simulink model "simulacija"  (R2015a)
settings: Solver=ode45  StartTime=0.0  StopTime=500  RelTol=1e-3
values from neighbouring files (symbols this model uses):
  C = C_r/m    (= 5.618808)    [parametri.m]
  K = 2*n*R_t/R    [parametri.m]
  R = R_r/m    [parametri.m]
  R_s1 = 1/(alfa_vaz*2*(a+b)*L/m)    (= 89.1265597148)    [parametri.m]
  R_s2 = 1/(alfa_vaz*a*b)    (= 1014.19878296)    [parametri.m]
  teta_k = 70    [parametri.m]
  teta_vaz = 30    [parametri.m]
settings Model: Creator=zracenje  LastModifiedBy=Danijel
settings DebuggingCC: UnderspecifiedInitializationDetection=Classic  MergeDetectMultiDrivingBlocksExec=none  SolverPrmCheckMsg=warning

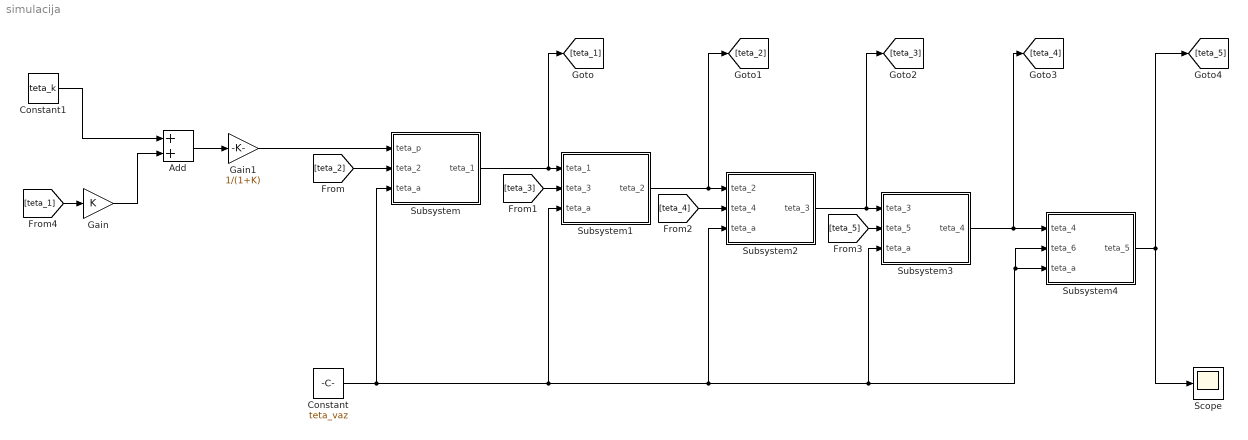
== system simulacija ==
  Add : Sum
  Constant : Constant  Value=teta_vaz
  Constant1 : Constant  Value=teta_k
  Gain : Gain  Gain=K
  Gain1 : Gain  Gain=1/(1+K)
  Scope : Scope
      settings: TimeRange=500  YMin=30  YMax=65
  Subsystem : Subsystem
  Subsystem1 : Subsystem
  Subsystem2 : Subsystem
  Subsystem3 : Subsystem
  Subsystem4 : Subsystem
  wires:
  Subsystem/1(teta_1) -> [teta_1], Subsystem1/1(teta_1)
  Subsystem1/1(teta_2) -> [teta_2], Subsystem2/1(teta_2)
  Subsystem2/1(teta_3) -> [teta_3], Subsystem3/1(teta_3)
  Subsystem3/1(teta_4) -> [teta_4], Subsystem4/1(teta_4)
  Constant/1 -> Subsystem1/3("teta_a "), Subsystem2/3("teta_a "), Subsystem3/3("teta_a "), Subsystem4/2(teta_6), Subsystem4/3("teta_a "), Subsystem/3("teta_a ")
  Subsystem4/1(teta_5) -> [teta_5], Scope/1
  [teta_2] -> Subsystem/2(teta_2)
  [teta_3] -> Subsystem1/2(teta_3)
  [teta_4] -> Subsystem2/2(teta_4)
  [teta_5] -> Subsystem3/2(teta_5)
  Constant1/1 -> Add/1
  Gain/1 -> Add/2
  [teta_1] -> Gain/1
  Add/1 -> Gain1/1
  Gain1/1 -> Subsystem/1(teta_p)

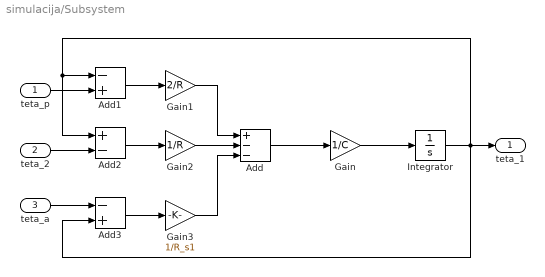
== system simulacija/Subsystem ==
  teta_p : Inport
  teta_2 : Inport  Port=2
  "teta_a " : Inport  Port=3
  Add : Sum  Inputs=+--
  Add1 : Sum  Inputs=-+
  Add2 : Sum  Inputs=+-
  Add3 : Sum  Inputs=-+
  Gain : Gain  Gain=1/C
  Gain1 : Gain  Gain=2/R
  Gain2 : Gain  Gain=1/R
  Gain3 : Gain  Gain=1/R_s1
  Integrator : Integrator  InitialCondition=teta_vaz
  teta_1 : Outport
  wires:
  Add/1 -> Gain/1
  Gain/1 -> Integrator/1
  Integrator/1 -> Add3/2, Add1/1, Add2/1, teta_1/1
  Add1/1 -> Gain1/1
  Gain1/1 -> Add/1
  Gain2/1 -> Add/2
  Add2/1 -> Gain2/1
  Gain3/1 -> Add/3
  Add3/1 -> Gain3/1
  "teta_a "/1 -> Add3/1
  teta_2/1 -> Add2/2
  teta_p/1 -> Add1/2

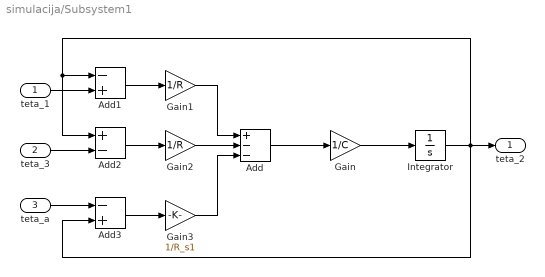
== system simulacija/Subsystem1 ==
  teta_1 : Inport
  teta_3 : Inport  Port=2
  "teta_a " : Inport  Port=3
  Add : Sum  Inputs=+--
  Add1 : Sum  Inputs=-+
  Add2 : Sum  Inputs=+-
  Add3 : Sum  Inputs=-+
  Gain : Gain  Gain=1/C
  Gain1 : Gain  Gain=1/R
  Gain2 : Gain  Gain=1/R
  Gain3 : Gain  Gain=1/R_s1
  Integrator : Integrator  InitialCondition=teta_vaz
  teta_2 : Outport
  wires:
  Add/1 -> Gain/1
  Gain/1 -> Integrator/1
  Integrator/1 -> Add3/2, Add1/1, Add2/1, teta_2/1
  Add1/1 -> Gain1/1
  Gain1/1 -> Add/1
  Gain2/1 -> Add/2
  Add2/1 -> Gain2/1
  Gain3/1 -> Add/3
  Add3/1 -> Gain3/1
  "teta_a "/1 -> Add3/1
  teta_3/1 -> Add2/2
  teta_1/1 -> Add1/2

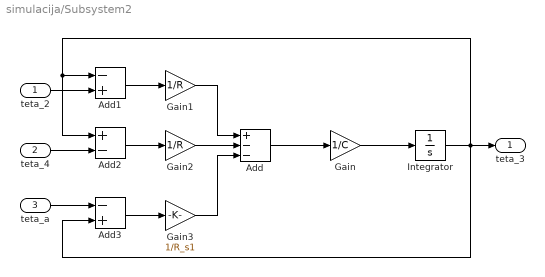
== system simulacija/Subsystem2 ==
  teta_2 : Inport
  teta_4 : Inport  Port=2
  "teta_a " : Inport  Port=3
  Add : Sum  Inputs=+--
  Add1 : Sum  Inputs=-+
  Add2 : Sum  Inputs=+-
  Add3 : Sum  Inputs=-+
  Gain : Gain  Gain=1/C
  Gain1 : Gain  Gain=1/R
  Gain2 : Gain  Gain=1/R
  Gain3 : Gain  Gain=1/R_s1
  Integrator : Integrator  InitialCondition=teta_vaz
  teta_3 : Outport
  wires:
  Add/1 -> Gain/1
  Gain/1 -> Integrator/1
  Integrator/1 -> Add3/2, Add1/1, Add2/1, teta_3/1
  Add1/1 -> Gain1/1
  Gain1/1 -> Add/1
  Gain2/1 -> Add/2
  Add2/1 -> Gain2/1
  Gain3/1 -> Add/3
  Add3/1 -> Gain3/1
  "teta_a "/1 -> Add3/1
  teta_4/1 -> Add2/2
  teta_2/1 -> Add1/2

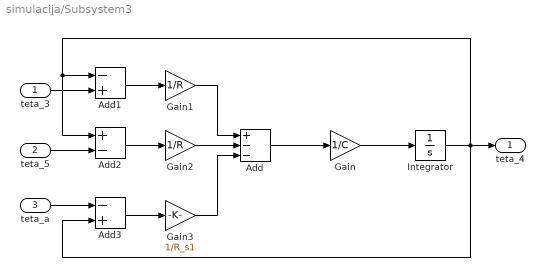
== system simulacija/Subsystem3 ==
  teta_3 : Inport
  teta_5 : Inport  Port=2
  "teta_a " : Inport  Port=3
  Add : Sum  Inputs=+--
  Add1 : Sum  Inputs=-+
  Add2 : Sum  Inputs=+-
  Add3 : Sum  Inputs=-+
  Gain : Gain  Gain=1/C
  Gain1 : Gain  Gain=1/R
  Gain2 : Gain  Gain=1/R
  Gain3 : Gain  Gain=1/R_s1
  Integrator : Integrator  InitialCondition=teta_vaz
  teta_4 : Outport
  wires:
  Add/1 -> Gain/1
  Gain/1 -> Integrator/1
  Integrator/1 -> Add3/2, Add1/1, Add2/1, teta_4/1
  Add1/1 -> Gain1/1
  Gain1/1 -> Add/1
  Gain2/1 -> Add/2
  Add2/1 -> Gain2/1
  Gain3/1 -> Add/3
  Add3/1 -> Gain3/1
  "teta_a "/1 -> Add3/1
  teta_5/1 -> Add2/2
  teta_3/1 -> Add1/2

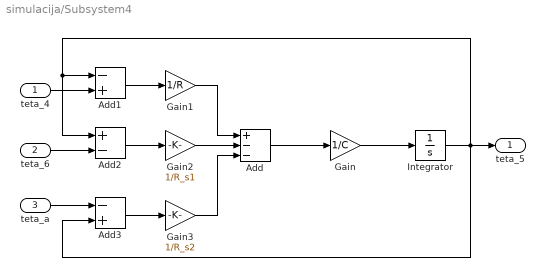
== system simulacija/Subsystem4 ==
  teta_4 : Inport
  teta_6 : Inport  Port=2
  "teta_a " : Inport  Port=3
  Add : Sum  Inputs=+--
  Add1 : Sum  Inputs=-+
  Add2 : Sum  Inputs=+-
  Add3 : Sum  Inputs=-+
  Gain : Gain  Gain=1/C
  Gain1 : Gain  Gain=1/R
  Gain2 : Gain  Gain=1/R_s1
  Gain3 : Gain  Gain=1/R_s2
  Integrator : Integrator  InitialCondition=teta_vaz
  teta_5 : Outport
  wires:
  Add/1 -> Gain/1
  Gain/1 -> Integrator/1
  Integrator/1 -> Add3/2, Add1/1, Add2/1, teta_5/1
  Add1/1 -> Gain1/1
  Gain1/1 -> Add/1
  Gain2/1 -> Add/2
  Add2/1 -> Gain2/1
  Gain3/1 -> Add/3
  Add3/1 -> Gain3/1
  "teta_a "/1 -> Add3/1
  teta_6/1 -> Add2/2
  teta_4/1 -> Add1/2
